simulink model "example_quadcopter_discrete"  (R2016a)
settings: Solver=VariableStepAuto  StartTime=0.0  StopTime=2.5  RelTol=1e-3
settings Model: Creator=Daniel  LastModifiedBy=mgreiff
settings DataIOCC: LimitDataPoints=on
settings DebuggingCC: AllowSymbolicDim=off
settings ModelReferenceCC: PropagateSignalLabelsOutOfModel=off
settings GRTTargetCC: GeneratePreprocessorConditionals=Use local settings

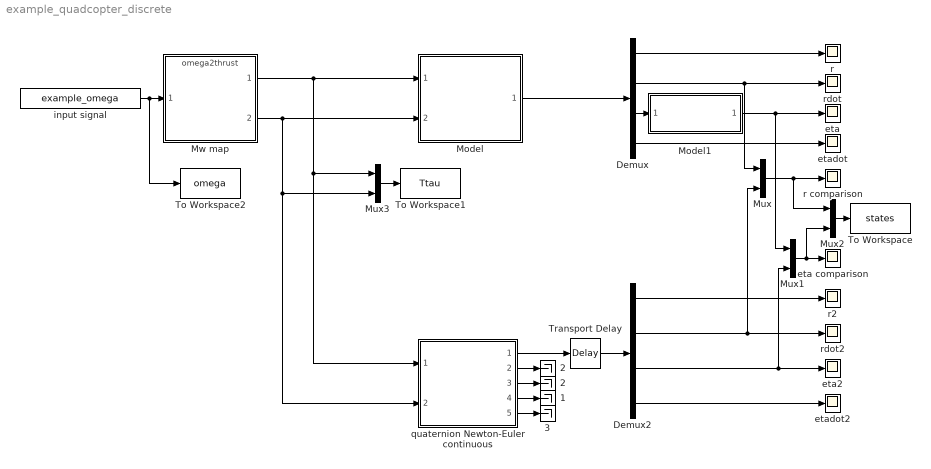
== system example_quadcopter_discrete ==
  "  2" : Terminator
  " 1" : Terminator
  " 2" : Terminator
  " 3" : Terminator
  Demux : Demux  Outputs=[3,3,4,3]
  Demux2 : Demux  Outputs=[3,3,3,3]
  Model : ModelReference  ModelNameDialog=quadcopter_model_d_NewtonEuler.mdl  SimulationMode=Normal  ModelReferenceVersion=1.308
  Model1 : ModelReference  ModelNameDialog=quaternion2euler.mdl  SimulationMode=Normal  ModelReferenceVersion=1.92
  Mux{,1..3} (4 alike) : Mux  Inputs=2
  Mw map : ModelReference  ModelNameDialog=omega2thrust.mdl  SimulationMode=Normal  ModelReferenceVersion=1.3
  To Workspace : ToWorkspace  VariableName=states  SaveFormat=Timeseries  SampleTime=-1
  To Workspace1 : ToWorkspace  VariableName=Ttau  SaveFormat=Timeseries  SampleTime=-1
  To Workspace2 : ToWorkspace  VariableName=omega  SaveFormat=Timeseries  SampleTime=-1
  Transport Delay : TransportDelay  DelayTime=1/60
  eta : Scope
  eta comparison : Scope
  eta2 : Scope
  etadot : Scope
  etadot2 : Scope
  input signal : FromFile  FileName=example_omega  SampleTime=0.0001  ExtrapolationBeforeFirstDataPoint=Hold first value
  quaternion Newton-Euler continuous : ModelReference  ModelNameDialog=quadcopter_model_c_NewtonEuler.mdl  SimulationMode=Normal  ModelReferenceVersion=1.320
  r : Scope
  r comparison : Scope
  r2 : Scope
  rdot : Scope
  rdot2 : Scope
  wires:
  input signal/1 -> To Workspace2/1, Mw map/1
  Demux/2 -> Mux/1, rdot/1
  Demux/1 -> r/1
  Demux/4 -> etadot/1
  Mw map/2 -> quaternion Newton-Euler continuous/2, Mux3/2, Model/2
  Mw map/1 -> Mux3/1, quaternion Newton-Euler continuous/1, Model/1
  quaternion Newton-Euler continuous/1 -> Transport Delay/1
  Demux2/2 -> Mux/2, rdot2/1
  Demux2/1 -> r2/1
  Demux2/4 -> etadot2/1
  Demux2/3 -> Mux1/2, eta2/1
  quaternion Newton-Euler continuous/3 -> "  2"/1
  quaternion Newton-Euler continuous/2 -> " 2"/1
  Mux/1 -> Mux2/1, r comparison/1
  Demux/3 -> Model1/1
  Model1/1 -> Mux1/1, eta/1
  quaternion Newton-Euler continuous/4 -> " 1"/1
  quaternion Newton-Euler continuous/5 -> " 3"/1
  Mux1/1 -> Mux2/2, eta comparison/1
  Model/1 -> Demux/1
  Transport Delay/1 -> Demux2/1
  Mux2/1 -> To Workspace/1
  Mux3/1 -> To Workspace1/1
